simulink model "CompareTo3"  (Simulink 9.0)
settings: Solver=FixedStepAuto  StartTime=0.0  StopTime=10.0  FixedStep=1.000000  RelTol=1e-3  EnableMultiTasking=on
libraries: simulink x9
settings Model: SuppressorTable=22 serialization::archive 11 0 6 0 0 0 0 0  Creator=arnaud  LastModifiedBy=hbourbou
settings DataIOCC: LimitDataPoints=on  SaveFormat=Structure
settings DebuggingCC: UnderspecifiedInitializationDetection=Simplified  MergeDetectMultiDrivingBlocksExec=error  SolverPrmCheckMsg=warning
settings GRTTargetCC: GeneratePreprocessorConditionals=Disable all
settings ConfigComp: CovSFcnEnable=off

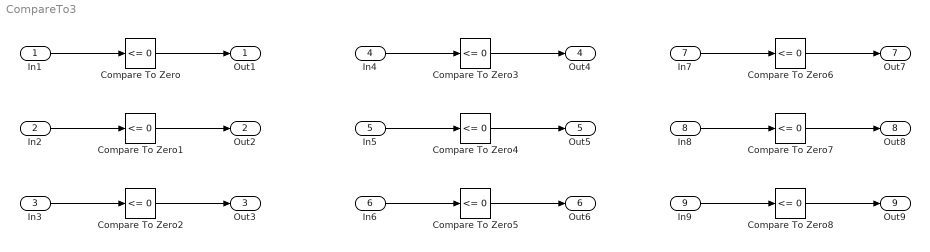
== system CompareTo3 ==
  In1 : Inport  OutDataTypeStr=double
  In2 : Inport  Port=2  OutDataTypeStr=int8
  In3 : Inport  Port=3  OutDataTypeStr=boolean
  In4 : Inport  Port=4  OutDataTypeStr=double  PortDimensions=3
  In5 : Inport  Port=5  OutDataTypeStr=int8  PortDimensions=3
  In6 : Inport  Port=6  OutDataTypeStr=boolean  PortDimensions=3
  In7 : Inport  Port=7  OutDataTypeStr=double  PortDimensions=[2 3]
  In8 : Inport  Port=8  OutDataTypeStr=int8  PortDimensions=[2 3]
  In9 : Inport  Port=9  OutDataTypeStr=boolean  PortDimensions=[2 3]
  Compare To Zero{,1..8} (9 alike) : simulink/Logic and Bit Operations/Compare To Zero  relop=<=  OutDataTypeStr=boolean
  Out1 : Outport
  Out2 : Outport  Port=2
  Out3 : Outport  Port=3
  Out4 : Outport  Port=4
  Out5 : Outport  Port=5
  Out6 : Outport  Port=6
  Out7 : Outport  Port=7
  Out8 : Outport  Port=8
  Out9 : Outport  Port=9
  wires:
  Compare To Zero/1 -> Out1/1
  In1/1 -> Compare To Zero/1
  Compare To Zero1/1 -> Out2/1
  In2/1 -> Compare To Zero1/1
  Compare To Zero2/1 -> Out3/1
  In3/1 -> Compare To Zero2/1
  Compare To Zero3/1 -> Out4/1
  In4/1 -> Compare To Zero3/1
  Compare To Zero4/1 -> Out5/1
  In5/1 -> Compare To Zero4/1
  Compare To Zero5/1 -> Out6/1
  In6/1 -> Compare To Zero5/1
  Compare To Zero6/1 -> Out7/1
  In7/1 -> Compare To Zero6/1
  Compare To Zero7/1 -> Out8/1
  In8/1 -> Compare To Zero7/1
  Compare To Zero8/1 -> Out9/1
  In9/1 -> Compare To Zero8/1
